simulink model "pump_simulator"  (R2020b)
settings: Solver=ode23t  StartTime=0.0  StopTime=sim_time  FixedStep=6.0  MaxStep=6.0  RelTol=1e-3
values from neighbouring files (symbols this model uses):
  bolus_size = 10    [insulin_pump.m]
  bolus_time = 3600*3    (= 10800)    [insulin_pump.m]
  damper_d1 = 5.0e4    (= 50000)    [insulin_pump.m]
  damper_d2 = 5    [insulin_pump.m]
  iis_area = pi*iis_diameter^2    (= 3.14159265359)    [insulin_pump.m]
  iis_elevation = 0    [insulin_pump.m]
  m_pulse_period = 3600 / n_pulses_per_hour    (= 180)    [insulin_pump.m]
  m_rotor_inertia = 0.051    [insulin_pump.m]
  m_volt = m_volt_nom    (= 3)    [insulin_pump.m]
  occ_area = iis_area    (= 3.14159265359)    [insulin_pump.m]
  occ_sw = 1    [insulin_pump.m]
  occ_tau = 2000    [insulin_pump.m]
  occ_time = s_locs(occ_idx)    [detect_occlusion.m]    (also in insulin_pump.m = 7200)
  piston_area = pi*reservoir_radius^2    [insulin_pump.m]
  piston_displacement_per_unit = U_per_ml / (piston_area)    [insulin_pump.m]
  piston_length = reservoir_len    (= 2.5)    [insulin_pump.m]
  pump_stop_time = 3600*6    (= 21600)    [insulin_pump.m]
  s_per_U = 60/flow_ml_min / 100    (= 12)    [insulin_pump.m]
  sim_time = 3600 * 10    (= 36000)    [insulin_pump.m]
  u_per_basal_pulse = basal_rate / n_pulses_per_hour    (= 0.05)    [insulin_pump.m]
libraries: fl_lib x38, nesl_utility x28, sh_lib x11, ee_lib x4, sdl_lib x3, simulink x1
(part 2 of 2)

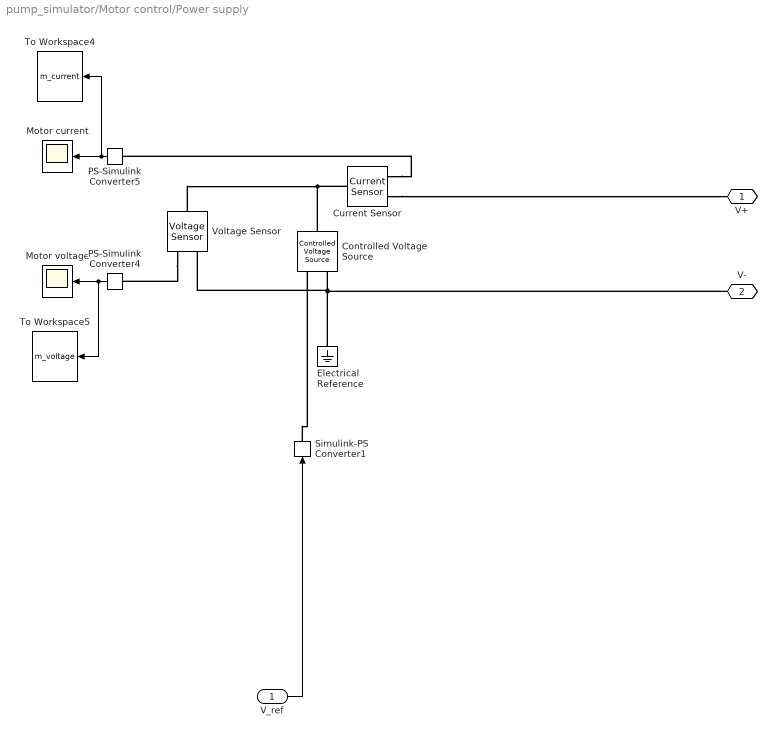
== system pump_simulator/Motor control/Power supply ==
  V_ref : Inport
  Controlled Voltage Source : fl_lib/Electrical/Electrical Sources/Controlled Voltage Source
  "Current Sensor " : fl_lib/Electrical/Electrical Sensors/Current Sensor
  "Electrical Reference " : fl_lib/Electrical/Electrical Elements/Electrical Reference
  Motor current : Scope
  Motor voltage : Scope
  PS-Simulink Converter4 : nesl_utility/PS-Simulink Converter  PhysicalDomain=network_engine_domain  SubClassName=ps_output  LeftPortType=input  RightPortType=output  PseudoPeriodic=off  Frequencies=[]  Unit=inherit  AffineConversion=off
  PS-Simulink Converter5 : nesl_utility/PS-Simulink Converter  PhysicalDomain=network_engine_domain  SubClassName=ps_output  LeftPortType=input  RightPortType=output  PseudoPeriodic=off  Frequencies=[]  Unit=inherit  AffineConversion=off
  Simulink-PS Converter1 : nesl_utility/Simulink-PS Converter  PhysicalDomain=network_engine_domain  SubClassName=ps_input  LeftPortType=input  RightPortType=output  PseudoPeriodic=off  Frequencies=[]  NoiseDistribution=none  NoiseParameters=[]  Unit=1  AffineConversion=off  FilteringAndDerivatives=filter  SimscapeFilterOrder=1  InputFilterTimeConstant=0.001  UdotUserProvided=0
  To Workspace4 : ToWorkspace  VariableName=m_current  SaveFormat=Timeseries  SampleTime=-1
  To Workspace5 : ToWorkspace  VariableName=m_voltage  SaveFormat=Timeseries  SampleTime=-1
  "Voltage Sensor " : fl_lib/Electrical/Electrical Sensors/Voltage Sensor
  V+ : PMIOPort  Side=Right
  V- : PMIOPort  Port=2  Side=Right
  wires:
  PS-Simulink Converter5/1 -> To Workspace4/1, Motor current/1
  V_ref/1 -> Simulink-PS Converter1/1
  PS-Simulink Converter4/1 -> To Workspace5/1, Motor voltage/1
  connections:
  "Electrical Reference "/LConn1 -- V-/RConn1 -- "Voltage Sensor "/RConn2 -- Controlled Voltage Source/RConn2
  "Current Sensor "/RConn2 -- V+/RConn1
  "Current Sensor "/LConn1 -- Controlled Voltage Source/LConn1 -- "Voltage Sensor "/LConn1
  "Voltage Sensor "/RConn1 -- PS-Simulink Converter4/LConn1
  "Current Sensor "/RConn1 -- PS-Simulink Converter5/LConn1
  Simulink-PS Converter1/RConn1 -- Controlled Voltage Source/RConn1
